simulink model "exp3"  (R2014b)
settings: Solver=ode45  StartTime=0.0  StopTime=10.0  RelTol=1e-3
settings Model: Creator=Ankit  LastModifiedBy=Ankit

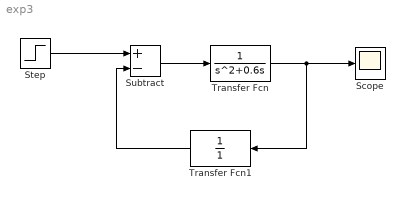
== system exp3 ==
  Scope : Scope
  Step : Step  Time=.1  Before=-2  SampleTime=0
  Subtract : Sum  Inputs=+-
  Transfer Fcn : TransferFcn  Denominator=[1 0.6 0]
  Transfer Fcn1 : TransferFcn  Denominator=[1]
  wires:
  Step/1 -> Subtract/1
  Transfer Fcn1/1 -> Subtract/2
  Subtract/1 -> Transfer Fcn/1
  Transfer Fcn/1 -> Scope/1, Transfer Fcn1/1
